simulink model "rhp_zero"  (R2015a)
settings: Solver=ode45  StartTime=0.0  StopTime=4  RelTol=1e-3
libraries: cstblocks x4
settings Model: Creator=Kripa95  LastModifiedBy=Kripa95

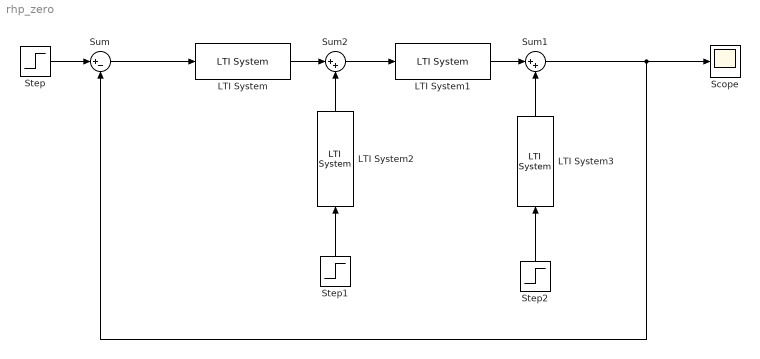
== system rhp_zero ==
  LTI System : cstblocks/LTI System  sys=con  IC=[]
  LTI System1 : cstblocks/LTI System  sys=g  IC=[]
  LTI System2 : cstblocks/LTI System  sys=d  IC=[]
  LTI System3 : cstblocks/LTI System  sys=ld  IC=[]
  Scope : Scope
      settings: YMin=-6  YMax=1
  Step : Step  After=15  SampleTime=0
  Step1 : Step  Time=3  SampleTime=0
  Step2 : Step  Time=2  SampleTime=0
  Sum : Sum  Inputs=|+-
  Sum1 : Sum  Inputs=|++
  Sum2 : Sum  Inputs=|++
  wires:
  LTI System1/1 -> Sum1/1
  Sum1/1 -> Sum/2, Scope/1
  LTI System3/1 -> Sum1/2
  Step2/1 -> LTI System3/1
  Step1/1 -> LTI System2/1
  Step/1 -> Sum/1
  LTI System/1 -> Sum2/1
  LTI System2/1 -> Sum2/2
  Sum/1 -> LTI System/1
  Sum2/1 -> LTI System1/1
